simulink model "linear_sim"  (R2024b)
settings: Solver=VariableStepAuto  StartTime=0.0  StopTime=10.0  MaxStep=1e-4  RelTol=1e-3
values from neighbouring files (symbols this model uses):
  K = -lqr(sys,Q,R,0)    [linear_model.m]
  K_pre = 1/dcgain(sys_cl(1,1))    [linear_model.m]
  V = 100    [linear_model.m]
undefined symbols (not defined in the file or in its folder): c_l_d, gaussian, ref_area, ref_length, rho, tau
libraries: simulink x4, aerolibactuator x1
settings Model: Creator=finnb  LastModifiedBy=finnb

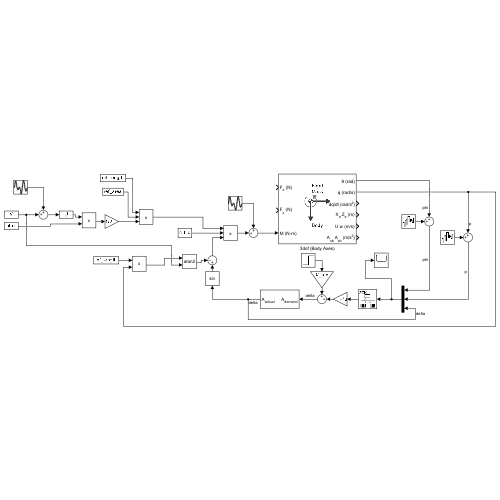
[thumbnail: Simulink's stored preview of the top-level diagram]
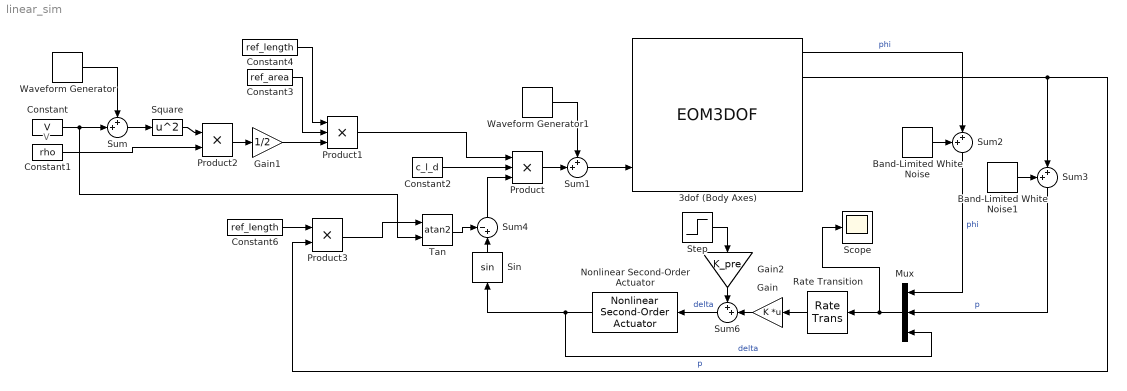
== system linear_sim ==
  note: V
  3dof (Body Axes) : EOM3DOF  v_ini=0  mass=100  Iyy=J  g=0
  Band-Limited White Noise : simulink/Sources/Band-Limited White Noise  Cov=[1e-8]  Ts=0.005  seed=[23341]
  Band-Limited White Noise1 : simulink/Sources/Band-Limited White Noise  Cov=[1e-6]  Ts=0.005  seed=[23341]
  Constant : Constant  Value=V
  Constant1 : Constant  Value=rho
  Constant2 : Constant  Value=c_l_d
  Constant3 : Constant  Value=ref_area
  Constant4 : Constant  Value=ref_length
  Constant6 : Constant  Value=ref_length
  Gain : Gain  Gain=K  Multiplication=Matrix(K*u)
  Gain1 : Gain  Gain=1/2
  Gain2 : Gain  Gain=K_pre
  Mux : Mux  Inputs=3
  Nonlinear Second-Order Actuator : aerolibactuator/Nonlinear Second-Order Actuator  wn_fin=1/tau  z_fin=0.9  fin_max=15*pi/180  fin_min=-15*pi/180  fin_maxrate=60/0.01*pi/180  fin_act_0=0  fin_act_vel=0
  Product : Product  Inputs=3
  Product1 : Product  Inputs=3
  Product2 : Product
  Product3 : Product
  Rate Transition : RateTransition  OutPortSampleTime=0.01
  Scope : Scope
  Sin : Trigonometry
  Square : Math  Operator=square
  Step : Step  SampleTime=0
  Sum{,1..3,6} (5 alike) : Sum  Inputs=++|
  Sum4 : Sum  Inputs=-+|
  Tan : Trigonometry  Operator=atan2
  Waveform Generator : simulink/Sources/Waveform Generator  OutMin=[]  OutMax=[]  OutDataTypeStr=double  SelectedSignal=1  Signals=gaussian(0,5,1)  BlockNames=MultiportSwitch_c1f80dc3b1be420  SampleTime=0.1
  Waveform Generator1 : simulink/Sources/Waveform Generator  OutMin=[]  OutMax=[]  OutDataTypeStr=double  SelectedSignal=1  Signals=gaussian(0.1,0.2,1)  BlockNames=MultiportSwitch_766c6aec0f6d441  SampleTime=0.1
  wires:
  Mux/1 -> Scope/1, Rate Transition/1
  Gain/1 -> Sum6/2
  3dof (Body Axes)/1 -> Sum2/2  "phi"
  3dof (Body Axes)/2 -> Sum3/2, Product3/2  "p"
  Constant/1 -> Tan/2, Sum/2
  Constant1/1 -> Product2/2
  Product/1 -> Sum1/2
  Sin/1 -> Sum4/2
  Constant2/1 -> Product/2
  Product1/1 -> Product/1
  Product2/1 -> Gain1/1
  Constant3/1 -> Product1/2
  Constant4/1 -> Product1/1
  Waveform Generator/1 -> Sum/1
  Sum/1 -> Square/1
  Sum1/1 -> 3dof (Body Axes)/3
  Waveform Generator1/1 -> Sum1/1
  Square/1 -> Product2/1
  Gain1/1 -> Product1/3
  Sum2/1 -> Mux/1  "phi"
  Band-Limited White Noise/1 -> Sum2/1
  Band-Limited White Noise1/1 -> Sum3/1
  Sum3/1 -> Mux/2  "p"
  Constant6/1 -> Product3/1
  Sum4/1 -> Product/3
  Tan/1 -> Sum4/1
  Product3/1 -> Tan/1
  Gain2/1 -> Sum6/1
  Step/1 -> Gain2/1
  Rate Transition/1 -> Gain/1
  Nonlinear Second-Order Actuator/1 -> Mux/3, Sin/1  "delta"
  Sum6/1 -> Nonlinear Second-Order Actuator/1  "delta"
